simulink model "mdl_offset_PWM_test1"  (R2022b)
settings: Solver=ode3  StartTime=0.0  StopTime=0.6  FixedStep=1e-6  RelTol=1e-3  EnableMultiTasking=on
libraries: spsTriangleGeneratorLib x2, spsDCVoltageSourceLib x1, spsGroundLib x1, spsPermanentMagnetSynchronousMachineLib x1, simulink x1, spsThreePhaseVIMeasurementLib x1, spsUniversalBridgeLib x1, spspowerguiLib x1
settings Model: Creator=jack  LastModifiedBy=jackyeh
settings DebuggingCC: SolverPrmCheckMsg=warning  StateNameClashWarn=warning

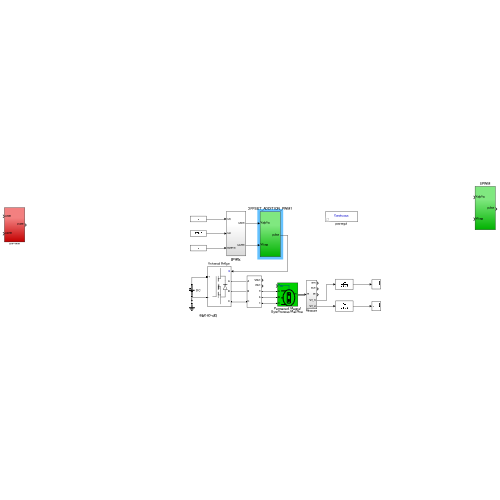
[thumbnail: Simulink's stored preview of the top-level diagram]
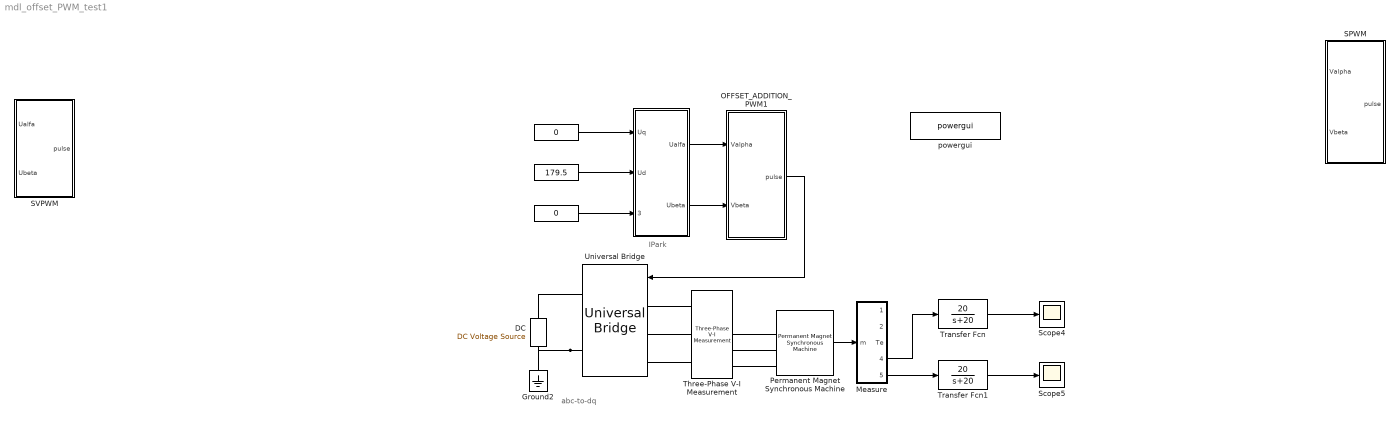
== system mdl_offset_PWM_test1 ==
  note: abc-to-dq
  note: IPark
  "  " : Constant  Value=0
  "   " : Constant  Value=179.5
  "     " : Subsystem
  "       " : Constant  Value=0
  "DC " : spsDCVoltageSourceLib/DC Voltage Source  Amplitude=311  Measurements=None
  Ground2 : spsGroundLib/Ground  LConnTagsString=a
  Measure : Subsystem
  OFFSET_ADDITION_PWM1 : Subsystem
  "Permanent Magnet Synchronous Machine " : spsPermanentMagnetSynchronousMachineLib/Permanent Magnet Synchronous Machine  NbPhases=3  FluxDistribution=Sinusoidal  RotorType=Salient-pole  MechanicalLoad=Torque Tm  PresetModel=No  ShowDetailedParameters=on  MeasurementBus=off  Resistance=1.2  Inductance=8.5e-3  dqInductances=[5.7e-3, 5.7e-3]  La=5.7e-3  MachineConstant=Flux linkage established by magnets (V.s)  Flux=0.03  VoltageCst=10.8828  TorqueCst=0.09  Flat=120  Mechanical="[0.00016  0 2]"  PolePairs=4  InitialConditions=[0,0, 0,0]  InitialConditions5ph=[0 0 0 0 0 0]  RefAngle=Aligned with phase A axis (original Park)  IterativeDiscreteModel=Trapezoidal non iterative  TsBlock=-1  TsPowergui=0
  SPWM : Subsystem
  SVPWM : Subsystem
  Scope4 : Scope
  Scope5 : Scope
  Three-Phase V-I Measurement : spsThreePhaseVIMeasurementLib/Three-Phase V-I Measurement  VoltageMeasurement=phase-to-phase  SetLabelV=off  LabelV=Vabc  Vpu=off  VpuLL=off  CurrentMeasurement=yes  SetLabelI=off  LabelI=Iabc  Ipu=off  Pbase=100e6  Vbase=500e3  OutputType=Complex  PhasorSimulation=off  PSBequivalent=0
  Transfer Fcn : TransferFcn  Numerator=[20]  Denominator=[1 20]
  Transfer Fcn1 : TransferFcn  Numerator=[20]  Denominator=[1 20]
  "Universal Bridge " : spsUniversalBridgeLib/Universal Bridge  Arms=3  SnubberResistance=1e5  SnubberCapacitance=inf  Device=MOSFET / Diodes  Ron=1e-3  Lon=0  ForwardVoltages="[  0  0  ]"  ForwardVoltage=0  GTOparameters=[ 10e-6 , 20e-6 ]  IGBTparameters=[ 1e-6 , 2e-6 ]  Measurements=None  Measurements_2=None  converterType=Rectifier
  powergui : spspowerguiLib/powergui  Priority=1  SimulationMode=Continuous  SampleTime=50e-6  frequency=60  Iterations=50  frequencyindice=0  Pbase=100e6  ErrMax=1e-4  UnitsV=kV  UnitsW=MW  buscounter=0  FunctionMessages=off  echomessages=off  EnableUseOfTLC=off  CurrentSourceSwitches=off  DisableSnubberDevices=off  DisableRonSwitches=off  DisableVfSwitches=off  DisplayEquations=off  AutomaticDiscreteSolvers=off  SolverType=Tustin/Backward Euler (TBE)  Interpol=off  ExternalGateDelay=off  methode=off  Ts=100  x0status=blocks  SPID=off  SwTol=0  HookPort=off  NonlinearTolerance=1e-4  nMaxIteration=100  ContinueOnMaxIteration=off  RestoreLinks=warning  ResistiveCurrentMeasurement=off  Frange=[0:2:500]  Ylog=off  Xlog=on  ShowGrid=off  save=off  variable=ZData  structure=0  ZoomFFT=off  StartTime=0.0  cycles=1  DisplayStyle=1  fundamental=60  FreqAxis=off  MaxFrequency=1000  frequencyindicesteady=1  RmsSteady=1  display=off
  wires:
  OFFSET_ADDITION_PWM1/1(pulse) -> "Universal Bridge "/1
  "     "/1(Ualfa) -> OFFSET_ADDITION_PWM1/1(Valpha)
  "     "/2(Ubeta) -> OFFSET_ADDITION_PWM1/2(Vbeta)
  "  "/1 -> "     "/1(Uq)
  "   "/1 -> "     "/2(Ud)
  "       "/1 -> "     "/3(thetma)
  "Permanent Magnet Synchronous Machine "/1 -> Measure/1(m)
  Measure/4(Vs_q) -> Transfer Fcn/1
  Measure/5(Vs_d) -> Transfer Fcn1/1
  Transfer Fcn/1 -> Scope4/1
  Transfer Fcn1/1 -> Scope5/1
  connections:
  "Universal Bridge "/RConn2 -- Ground2/LConn1 -- "DC "/LConn1
  "Universal Bridge "/LConn1 -- Three-Phase V-I Measurement/LConn1
  "Universal Bridge "/LConn3 -- Three-Phase V-I Measurement/LConn3
  Three-Phase V-I Measurement/RConn3 -- "Permanent Magnet Synchronous Machine "/LConn3
  Three-Phase V-I Measurement/RConn1 -- "Permanent Magnet Synchronous Machine "/LConn1
  Three-Phase V-I Measurement/RConn2 -- "Permanent Magnet Synchronous Machine "/LConn2
  "Universal Bridge "/RConn1 -- "DC "/RConn1
  "Universal Bridge "/LConn2 -- Three-Phase V-I Measurement/LConn2

== system mdl_offset_PWM_test1/      ==
  Uq : Inport
  Ud : Inport  Port=2
  thetma : Inport  Port=3
  Fcn : Fcn  Expr=cos(u[3])*u[2]-sin(u[3])*u[1]
  Fcn1 : Fcn  Expr=sin(u[3])*u[2]+cos(u[3])*u[1]
  Mux : Mux  Inputs=3
  Ualfa : Outport
  Ubeta : Outport  Port=2
  wires:
  Uq/1 -> Mux/1
  Ud/1 -> Mux/2
  thetma/1 -> Mux/3
  Mux/1 -> Fcn/1, Fcn1/1
  Fcn/1 -> Ualfa/1
  Fcn1/1 -> Ubeta/1

== system mdl_offset_PWM_test1/Measure ==
  m : Inport
  Bus Selector1 : BusSelector  OutputSignals=Rotor speed wm (rad/s),Rotor angle thetam (rad),Electromagnetic torque Te (N*m),Stator voltage Vs_q (V),Stator voltage Vs_d (V)
  wm : Outport
  The : Outport  Port=2
  Te : Outport  Port=3
  Vs_q : Outport  Port=4
  Vs_d : Outport  Port=5
  wires:
  Bus Selector1/2 -> The/1  "<Rotor angle thetam (rad)>"
  Bus Selector1/3 -> Te/1  "<Electromagnetic torque Te (N*m)>"
  m/1 -> Bus Selector1/1
  Bus Selector1/1 -> wm/1  "<Rotor speed wm (rad/s)>"
  Bus Selector1/4 -> Vs_q/1  "<Stator voltage Vs_q (V)>"
  Bus Selector1/5 -> Vs_d/1  "<Stator voltage Vs_d (V)>"

== system mdl_offset_PWM_test1/OFFSET_ADDITION_PWM1 ==
  Valpha : Inport
  Vbeta : Inport  Port=2
  Vdc/1.732 : Constant  Value=179.5
  inv_clarke : Subsystem
  offset_addition_SPWM : Subsystem
      settings: PortSchema="{\"entries\":[{\"content\":{\"sides\":[{\"content\":{\"connectorIds\":[\"In1\",\"In2\",\"In3\"]},\"type\":\"ConnectorPlacement.EquallySpacedRectSide\",\"uuid\":\"bd7bea3a-7add-49ec-8b52-f68dbb33beea\"},{\"content\":{\"connectorIds\":[\"Out1\"],\"side\":\"RIGHT\"},\"type\":\"ConnectorPlacement.EquallySpacedRectSide\",\"uuid\":\"aa5e81bc-27af-49d7-8d73-7e78ac021e04\"},{\"content\":{\"connectorIds\":[\"In4\"],\"side\":\"TOP\"},\"type\":\"ConnectorPlacement.EquallySpacedRectSide\",\"uuid\":\"5bcd18e6-6f27-4bab-991b-2041f8ef0a25\"}]},\"type\":\"ConnectorPlacement.EquallySpacedConnector\",\"uuid\":\"27ed4ada-ba8b-4440-bbdb-1c3a657b0505\"}],\"packageUris\":[\"http://schema.mathworks.com/mf0/Connector/R2020b\"],\"version\":\"1.0\"}"
  pulse : Outport
  wires:
  Valpha/1 -> inv_clarke/1(f_alpha)
  Vbeta/1 -> inv_clarke/2(f_beta)
  inv_clarke/1(fa) -> offset_addition_SPWM/1(vas)
  inv_clarke/2(fb) -> offset_addition_SPWM/2(vbs)
  inv_clarke/3(fc) -> offset_addition_SPWM/3(vcs)
  offset_addition_SPWM/1(g) -> pulse/1
  Vdc/1.732/1 -> offset_addition_SPWM/4(v_mag)

== system mdl_offset_PWM_test1/SPWM ==
  Valpha : Inport
  Vbeta : Inport  Port=2
  SPWM : Subsystem
      settings: PortSchema="{\"entries\":[{\"content\":{\"sides\":[{\"content\":{\"connectorIds\":[\"In1\",\"In2\",\"In3\"]},\"type\":\"ConnectorPlacement.EquallySpacedRectSide\",\"uuid\":\"2e80e29a-e7ca-4bee-8f3b-5f9ffed0b982\"},{\"content\":{\"connectorIds\":[\"Out1\"],\"side\":\"RIGHT\"},\"type\":\"ConnectorPlacement.EquallySpacedRectSide\",\"uuid\":\"0c6270c9-1844-47ee-a65a-a4a71ede4f1c\"},{\"content\":{\"connectorIds\":[\"In4\"],\"side\":\"TOP\"},\"type\":\"ConnectorPlacement.EquallySpacedRectSide\",\"uuid\":\"66204f8a-7778-4eb4-8d19-bce1483f6917\"}]},\"type\":\"ConnectorPlacement.EquallySpacedConnector\",\"uuid\":\"7fb70670-52e1-41c4-9c5d-64b5a697f5ed\"}],\"packageUris\":[\"http://schema.mathworks.com/mf0/Connector/R2020b\"],\"version\":\"1.0\"}"
  Vdc/2 : Constant  Value=155
  inv_clarke : Subsystem
  pulse : Outport
  wires:
  Valpha/1 -> inv_clarke/1(f_alpha)
  Vbeta/1 -> inv_clarke/2(f_beta)
  inv_clarke/1(fa) -> SPWM/1(vas)
  inv_clarke/2(fb) -> SPWM/2(vbs)
  inv_clarke/3(fc) -> SPWM/3(vcs)
  SPWM/1(g) -> pulse/1
  Vdc/2/1 -> SPWM/4(v_mag)

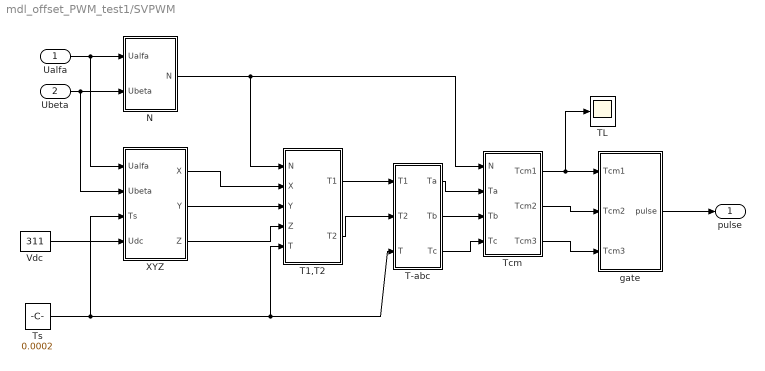
== system mdl_offset_PWM_test1/SVPWM ==
  Ualfa : Inport
  Ubeta : Inport  Port=2
  N : Subsystem
  T-abc : Subsystem
  T1,T2 : Subsystem
  TL : Scope
  Tcm : Subsystem
  Ts : Constant  Value=0.0002  SampleTime=-1
  Vdc : Constant  Value=311
  XYZ : Subsystem
  gate : Subsystem
  pulse : Outport
  wires:
  Tcm/1(Tcm1) -> gate/1(Tcm1), TL/1
  T-abc/2(Tb) -> Tcm/3(Tb)
  T-abc/1(Ta) -> Tcm/2(Ta)
  T-abc/3(Tc) -> Tcm/4(Tc)
  T1,T2/1(T1) -> T-abc/1(T1)
  T1,T2/2(T2) -> T-abc/2(T2)
  XYZ/2(Y) -> T1,T2/3(Y)
  XYZ/1(X) -> T1,T2/2(X)
  XYZ/3(Z) -> T1,T2/4(Z)
  N/1(N) -> T1,T2/1(N), Tcm/1(N)
  Ts/1 -> T1,T2/5(T), T-abc/3(T), XYZ/3(Ts)
  gate/1(pulse) -> pulse/1
  Ualfa/1 -> N/1(Ualfa), XYZ/1(Ualfa)
  Ubeta/1 -> N/2(Ubeta), XYZ/2(Ubeta)
  Vdc/1 -> XYZ/4(Udc)
  Tcm/2(Tcm2) -> gate/2(Tcm2)
  Tcm/3(Tcm3) -> gate/3(Tcm3)

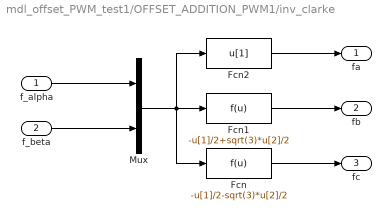
== system mdl_offset_PWM_test1/OFFSET_ADDITION_PWM1/inv_clarke ==
  f_alpha : Inport
  f_beta : Inport  Port=2
  Fcn : Fcn  Expr=-u[1]/2-sqrt(3)*u[2]/2
  Fcn1 : Fcn  Expr=-u[1]/2+sqrt(3)*u[2]/2
  Fcn2 : Fcn  Expr=u[1]
  Mux : Mux  Inputs=2
  fa : Outport
  fb : Outport  Port=2
  fc : Outport  Port=3
  wires:
  Mux/1 -> Fcn2/1, Fcn1/1, Fcn/1
  f_alpha/1 -> Mux/1
  f_beta/1 -> Mux/2
  Fcn2/1 -> fa/1
  Fcn1/1 -> fb/1
  Fcn/1 -> fc/1

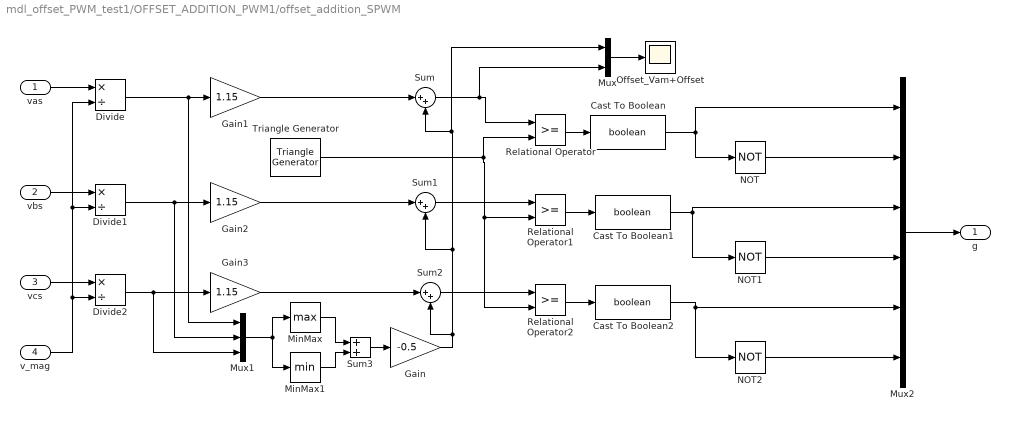
== system mdl_offset_PWM_test1/OFFSET_ADDITION_PWM1/offset_addition_SPWM ==
  vas : Inport
  vbs : Inport  Port=2
  vcs : Inport  Port=3
  v_mag : Inport  Port=4
  Cast To Boolean : DataTypeConversion  OutDataTypeStr=boolean  SaturateOnIntegerOverflow=off  RndMeth=Floor
  Cast To Boolean1 : DataTypeConversion  OutDataTypeStr=boolean  SaturateOnIntegerOverflow=off  RndMeth=Floor
  Cast To Boolean2 : DataTypeConversion  OutDataTypeStr=boolean  SaturateOnIntegerOverflow=off  RndMeth=Floor
  Divide : Product  Inputs=*/
  Divide1 : Product  Inputs=*/
  Divide2 : Product  Inputs=*/
  Gain : Gain  Gain=-0.5
  Gain1 : Gain  Gain=1.15
  Gain2 : Gain  Gain=1.15
  Gain3 : Gain  Gain=1.15
  MinMax : MinMax  Function=max
  MinMax1 : MinMax
  Mux : Mux  Inputs=2
  Mux1 : Mux  Inputs=3
  Mux2 : Mux  Inputs=6
  NOT : Logic  Operator=NOT  IconShape=distinctive  AllPortsSameDT=off  OutDataTypeStr=boolean
  NOT1 : Logic  Operator=NOT  IconShape=distinctive  AllPortsSameDT=off  OutDataTypeStr=boolean
  NOT2 : Logic  Operator=NOT  IconShape=distinctive  AllPortsSameDT=off  OutDataTypeStr=boolean
  Offset_Vam+Offset : Scope
  Relational Operator : RelationalOperator  OutDataTypeStr=boolean  RndMeth=Simplest  InputSameDT=off
  Relational Operator1 : RelationalOperator  OutDataTypeStr=boolean  RndMeth=Simplest  InputSameDT=off
  Relational Operator2 : RelationalOperator  OutDataTypeStr=boolean  RndMeth=Simplest  InputSameDT=off
  Sum : Sum  Inputs=|++
  Sum1 : Sum  Inputs=|++
  Sum2 : Sum  Inputs=|++
  Sum3 : Sum
  Triangle Generator : spsTriangleGeneratorLib/Triangle Generator  Freq=10000  Phase=90  Ts=0
  g : Outport
  wires:
  NOT/1 -> Mux2/2
  Relational Operator/1 -> Cast To Boolean/1
  Cast To Boolean/1 -> Mux2/1, NOT/1
  Triangle Generator/1 -> Relational Operator2/2, Relational Operator1/2, Relational Operator/2
  Relational Operator1/1 -> Cast To Boolean1/1
  Cast To Boolean1/1 -> Mux2/3, NOT1/1
  Relational Operator2/1 -> Cast To Boolean2/1
  NOT2/1 -> Mux2/6
  Cast To Boolean2/1 -> Mux2/5, NOT2/1
  Sum/1 -> Mux/2, Relational Operator/1
  Sum1/1 -> Relational Operator1/1
  Sum2/1 -> Relational Operator2/1
  Gain/1 -> Sum2/2, Sum1/2, Mux/1, Sum/2
  Mux1/1 -> MinMax1/1, MinMax/1
  MinMax/1 -> Sum3/1
  MinMax1/1 -> Sum3/2
  Sum3/1 -> Gain/1
  Mux/1 -> Offset_Vam+Offset/1
  vas/1 -> Divide/1
  v_mag/1 -> Divide/2, Divide1/2, Divide2/2
  vbs/1 -> Divide1/1
  vcs/1 -> Divide2/1
  Divide/1 -> Mux1/1, Gain1/1
  Divide1/1 -> Mux1/2, Gain2/1
  Divide2/1 -> Mux1/3, Gain3/1
  NOT1/1 -> Mux2/4
  Mux2/1 -> g/1
  Gain1/1 -> Sum/1
  Gain2/1 -> Sum1/1
  Gain3/1 -> Sum2/1

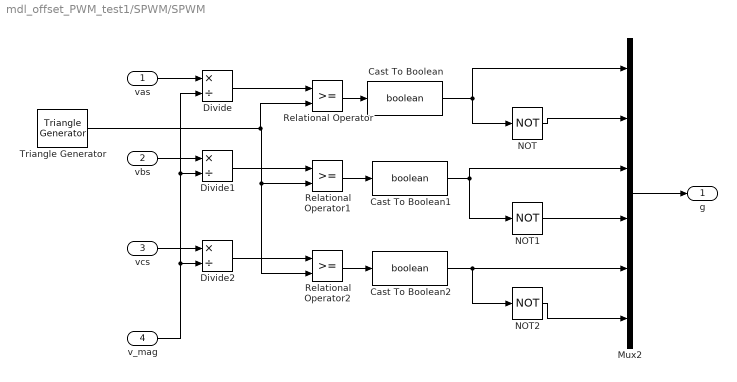
== system mdl_offset_PWM_test1/SPWM/SPWM ==
  vas : Inport
  vbs : Inport  Port=2
  vcs : Inport  Port=3
  v_mag : Inport  Port=4
  Cast To Boolean : DataTypeConversion  OutDataTypeStr=boolean  SaturateOnIntegerOverflow=off  RndMeth=Floor
  Cast To Boolean1 : DataTypeConversion  OutDataTypeStr=boolean  SaturateOnIntegerOverflow=off  RndMeth=Floor
  Cast To Boolean2 : DataTypeConversion  OutDataTypeStr=boolean  SaturateOnIntegerOverflow=off  RndMeth=Floor
  Divide : Product  Inputs=*/
  Divide1 : Product  Inputs=*/
  Divide2 : Product  Inputs=*/
  Mux2 : Mux  Inputs=6
  NOT : Logic  Operator=NOT  IconShape=distinctive  AllPortsSameDT=off  OutDataTypeStr=boolean
  NOT1 : Logic  Operator=NOT  IconShape=distinctive  AllPortsSameDT=off  OutDataTypeStr=boolean
  NOT2 : Logic  Operator=NOT  IconShape=distinctive  AllPortsSameDT=off  OutDataTypeStr=boolean
  Relational Operator : RelationalOperator  OutDataTypeStr=boolean  RndMeth=Simplest  InputSameDT=off
  Relational Operator1 : RelationalOperator  OutDataTypeStr=boolean  RndMeth=Simplest  InputSameDT=off
  Relational Operator2 : RelationalOperator  OutDataTypeStr=boolean  RndMeth=Simplest  InputSameDT=off
  Triangle Generator : spsTriangleGeneratorLib/Triangle Generator  Freq=2e3  Phase=90  Ts=0
  g : Outport
  wires:
  NOT/1 -> Mux2/2
  Relational Operator2/1 -> Cast To Boolean2/1
  Triangle Generator/1 -> Relational Operator/2, Relational Operator2/2, Relational Operator1/2
  NOT1/1 -> Mux2/4
  Cast To Boolean/1 -> Mux2/1, NOT/1
  Relational Operator/1 -> Cast To Boolean/1
  Cast To Boolean1/1 -> Mux2/3, NOT1/1
  NOT2/1 -> Mux2/6
  Relational Operator1/1 -> Cast To Boolean1/1
  Cast To Boolean2/1 -> Mux2/5, NOT2/1
  Mux2/1 -> g/1
  vas/1 -> Divide/1
  vbs/1 -> Divide1/1
  vcs/1 -> Divide2/1
  v_mag/1 -> Divide2/2, Divide1/2, Divide/2
  Divide/1 -> Relational Operator/1
  Divide1/1 -> Relational Operator1/1
  Divide2/1 -> Relational Operator2/1

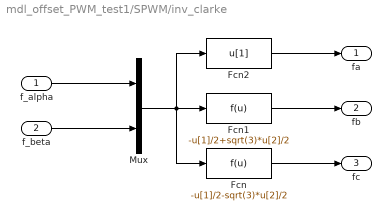
== system mdl_offset_PWM_test1/SPWM/inv_clarke ==
  f_alpha : Inport
  f_beta : Inport  Port=2
  Fcn : Fcn  Expr=-u[1]/2-sqrt(3)*u[2]/2
  Fcn1 : Fcn  Expr=-u[1]/2+sqrt(3)*u[2]/2
  Fcn2 : Fcn  Expr=u[1]
  Mux : Mux  Inputs=2
  fa : Outport
  fb : Outport  Port=2
  fc : Outport  Port=3
  wires:
  Mux/1 -> Fcn2/1, Fcn1/1, Fcn/1
  f_alpha/1 -> Mux/1
  f_beta/1 -> Mux/2
  Fcn2/1 -> fa/1
  Fcn1/1 -> fb/1
  Fcn/1 -> fc/1

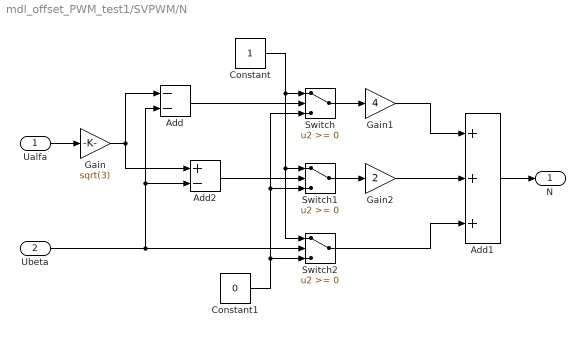
== system mdl_offset_PWM_test1/SVPWM/N ==
  Ualfa : Inport
  Ubeta : Inport  Port=2
  Add : Sum  Inputs=--
  Add1 : Sum  Inputs=+++
  Add2 : Sum  Inputs=+-
  Constant : Constant
  Constant1 : Constant  Value=0
  Gain : Gain  Gain=sqrt(3)
  Gain1 : Gain  Gain=4
  Gain2 : Gain  Gain=2
  Switch : Switch  SaturateOnIntegerOverflow=off  InputSameDT=off
  Switch1 : Switch  SaturateOnIntegerOverflow=off  InputSameDT=off
  Switch2 : Switch  SaturateOnIntegerOverflow=off  InputSameDT=off
  N : Outport
  wires:
  Ualfa/1 -> Gain/1
  Add1/1 -> N/1
  Switch/1 -> Gain1/1
  Add/1 -> Switch/2
  Gain/1 -> Add/1, Add2/1
  Ubeta/1 -> Switch2/2, Add/2, Add2/2
  Gain1/1 -> Add1/1
  Switch2/1 -> Add1/3
  Add2/1 -> Switch1/2
  Switch1/1 -> Gain2/1
  Gain2/1 -> Add1/2
  Constant/1 -> Switch2/1, Switch1/1, Switch/1
  Constant1/1 -> Switch/3, Switch1/3, Switch2/3

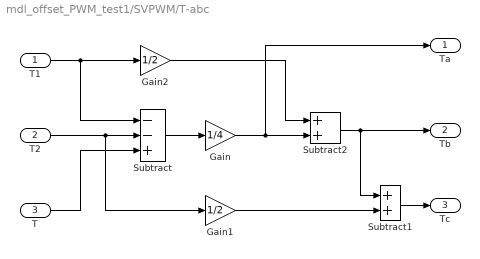
== system mdl_offset_PWM_test1/SVPWM/T-abc ==
  T1 : Inport
  T2 : Inport  Port=2
  T : Inport  Port=3
  Gain : Gain  Gain=1/4
  Gain1 : Gain  Gain=1/2
  Gain2 : Gain  Gain=1/2
  Subtract : Sum  Inputs=--+
  Subtract1 : Sum
  Subtract2 : Sum
  Ta : Outport
  Tb : Outport  Port=2
  Tc : Outport  Port=3
  wires:
  T2/1 -> Subtract/2, Gain1/1
  T1/1 -> Subtract/1, Gain2/1
  T/1 -> Subtract/3
  Subtract/1 -> Gain/1
  Gain/1 -> Ta/1, Subtract2/2
  Gain2/1 -> Subtract2/1
  Subtract2/1 -> Tb/1, Subtract1/1
  Subtract1/1 -> Tc/1
  Gain1/1 -> Subtract1/2

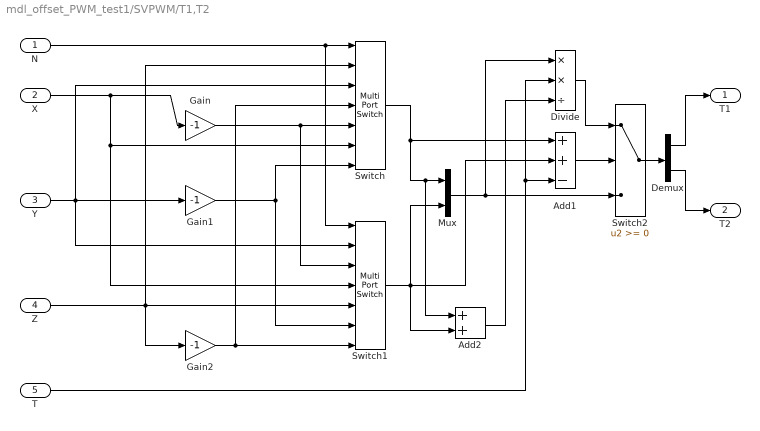
== system mdl_offset_PWM_test1/SVPWM/T1,T2 ==
  N : Inport
  X : Inport  Port=2
  Y : Inport  Port=3
  Z : Inport  Port=4
  T : Inport  Port=5
  Add1 : Sum  Inputs=++-
  Add2 : Sum
  Demux : Demux  Outputs=2
  Divide : Product  Inputs=**/
  Gain : Gain  Gain=-1
  Gain1 : Gain  Gain=-1
  Gain2 : Gain  Gain=-1
  Mux : Mux  Inputs=2
  Switch : MultiPortSwitch  Inputs=6  DiagnosticForDefault=None  SaturateOnIntegerOverflow=off  InputSameDT=off
  Switch1 : MultiPortSwitch  Inputs=6  DiagnosticForDefault=None  SaturateOnIntegerOverflow=off  InputSameDT=off
  Switch2 : Switch  SaturateOnIntegerOverflow=off  InputSameDT=off
  T1 : Outport
  T2 : Outport  Port=2
  wires:
  Y/1 -> Switch/3, Gain1/1, Switch1/2
  Z/1 -> Switch/2, Switch1/5, Gain2/1
  X/1 -> Gain/1, Switch1/4, Switch/6
  Gain/1 -> Switch/5, Switch1/3
  Gain2/1 -> Switch/4, Switch1/7
  Gain1/1 -> Switch1/6, Switch/7
  Switch/1 -> Add1/1, Mux/1, Add2/1
  Switch1/1 -> Mux/2, Add1/2, Add2/2
  Mux/1 -> Divide/1, Switch2/3
  Switch2/1 -> Demux/1
  Demux/1 -> T1/1
  Demux/2 -> T2/1
  Add1/1 -> Switch2/2
  T/1 -> Add1/3, Divide/2
  Divide/1 -> Switch2/1
  Add2/1 -> Divide/3
  N/1 -> Switch/1, Switch1/1

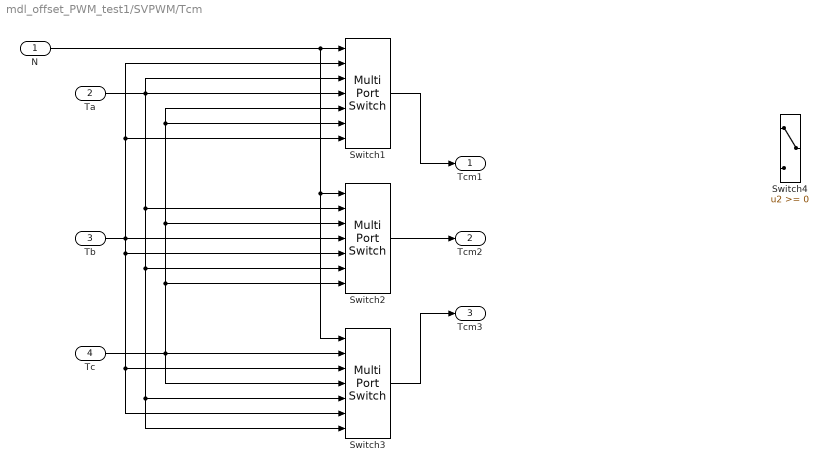
== system mdl_offset_PWM_test1/SVPWM/Tcm ==
  N : Inport
  Ta : Inport  Port=2
  Tb : Inport  Port=3
  Tc : Inport  Port=4
  Switch1 : MultiPortSwitch  Inputs=6  DiagnosticForDefault=None  SaturateOnIntegerOverflow=off  InputSameDT=off
  Switch2 : MultiPortSwitch  Inputs=6  DiagnosticForDefault=None  SaturateOnIntegerOverflow=off  InputSameDT=off
  Switch3 : MultiPortSwitch  Inputs=6  DiagnosticForDefault=None  SaturateOnIntegerOverflow=off  InputSameDT=off
  Switch4 : Switch  SaturateOnIntegerOverflow=off  InputSameDT=off
  Tcm1 : Outport
  Tcm2 : Outport  Port=2
  Tcm3 : Outport  Port=3
  wires:
  Switch2/1 -> Tcm2/1
  Switch3/1 -> Tcm3/1
  Switch1/1 -> Tcm1/1
  Tb/1 -> Switch2/4, Switch2/5, Switch3/3, Switch3/6, Switch1/2, Switch1/7
  Tc/1 -> Switch3/2, Switch3/4, Switch2/3, Switch1/5, Switch1/6, Switch2/7
  Ta/1 -> Switch1/4, Switch1/3, Switch2/2, Switch2/6, Switch3/5, Switch3/7
  N/1 -> Switch1/1, Switch2/1, Switch3/1

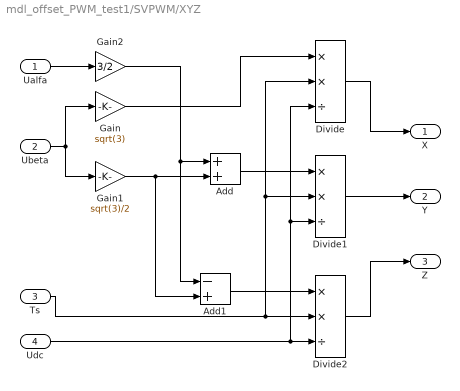
== system mdl_offset_PWM_test1/SVPWM/XYZ ==
  Ualfa : Inport
  Ubeta : Inport  Port=2
  Ts : Inport  Port=3
  Udc : Inport  Port=4
  Add : Sum
  Add1 : Sum  Inputs=-+
  Divide : Product  Inputs=**/
  Divide1 : Product  Inputs=**/
  Divide2 : Product  Inputs=**/
  Gain : Gain  Gain=sqrt(3)
  Gain1 : Gain  Gain=sqrt(3)/2
  Gain2 : Gain  Gain=3/2
  X : Outport
  Y : Outport  Port=2
  Z : Outport  Port=3
  wires:
  Divide1/1 -> Y/1
  Divide/1 -> X/1
  Divide2/1 -> Z/1
  Ts/1 -> Divide2/2, Divide1/2, Divide/2
  Udc/1 -> Divide2/3, Divide1/3, Divide/3
  Ubeta/1 -> Gain/1, Gain1/1
  Ualfa/1 -> Gain2/1
  Gain/1 -> Divide/1
  Add/1 -> Divide1/1
  Gain1/1 -> Add/2, Add1/2
  Gain2/1 -> Add1/1, Add/1
  Add1/1 -> Divide2/1

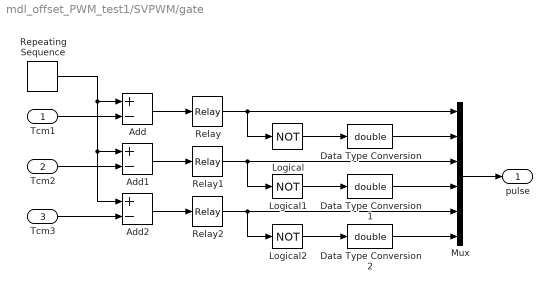
== system mdl_offset_PWM_test1/SVPWM/gate ==
  Tcm1 : Inport
  Tcm2 : Inport  Port=2
  Tcm3 : Inport  Port=3
  Add : Sum  Inputs=+-
  Add1 : Sum  Inputs=+-
  Add2 : Sum  Inputs=+-
  Data Type Conversion : DataTypeConversion  OutDataTypeStr=double  SaturateOnIntegerOverflow=off  RndMeth=Floor
  Data Type Conversion1 : DataTypeConversion  OutDataTypeStr=double  SaturateOnIntegerOverflow=off  RndMeth=Floor
  Data Type Conversion2 : DataTypeConversion  OutDataTypeStr=double  SaturateOnIntegerOverflow=off  RndMeth=Floor
  Logical : Logic  Operator=NOT  AllPortsSameDT=off  OutDataTypeStr=boolean
  Logical1 : Logic  Operator=NOT  AllPortsSameDT=off  OutDataTypeStr=boolean
  Logical2 : Logic  Operator=NOT  AllPortsSameDT=off  OutDataTypeStr=boolean
  Mux : Mux  Inputs=6
  Relay : Relay
  Relay1 : Relay
  Relay2 : Relay
  Repeating Sequence : simulink/Sources/Repeating Sequence  rep_seq_t=[0 0.00005 0.0001]  rep_seq_y=[0 0.0001 0]
  pulse : Outport
  wires:
  Tcm1/1 -> Add/2
  Tcm2/1 -> Add1/2
  Tcm3/1 -> Add2/2
  Repeating Sequence/1 -> Add2/1, Add1/1, Add/1
  Add2/1 -> Relay2/1
  Add1/1 -> Relay1/1
  Add/1 -> Relay/1
  Relay/1 -> Mux/1, Logical/1
  Relay1/1 -> Mux/3, Logical1/1
  Relay2/1 -> Mux/5, Logical2/1
  Data Type Conversion/1 -> Mux/2
  Logical/1 -> Data Type Conversion/1
  Data Type Conversion1/1 -> Mux/4
  Logical1/1 -> Data Type Conversion1/1
  Data Type Conversion2/1 -> Mux/6
  Logical2/1 -> Data Type Conversion2/1
  Mux/1 -> pulse/1
